simulink model "Task5AM"  (R2024a)
settings: Solver=VariableStepAuto  StartTime=0.0  StopTime=30  RelTol=1e-3
libraries: commanapbnd3 x1
settings Model: Creator=17760  LastModifiedBy=17760

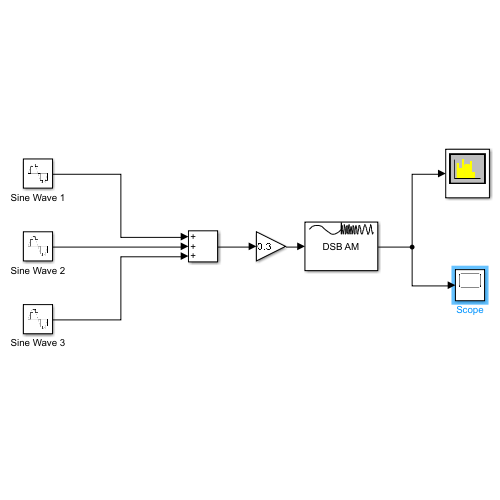
[thumbnail: Simulink's stored preview of the top-level diagram]
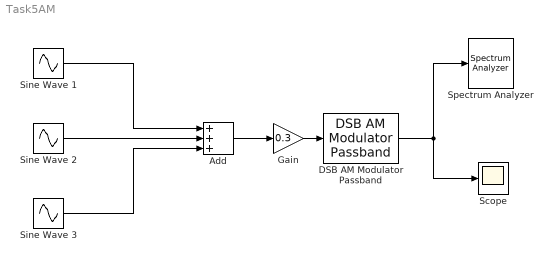
== system Task5AM ==
  Add : Sum  Inputs=+++
  DSB AM Modulator Passband : commanapbnd3/DSB AM Modulator Passband  Fc=300  Ph=0  Offset=1
  Gain : Gain  Gain=0.3
  Scope : Scope
  Sine Wave 1 : Sin  Amplitude=0.3  Frequency=2*pi*10  SampleTime=1/3000
  Sine Wave 2 : Sin  Amplitude=0.2  Frequency=2*pi*20  Phase=pi/6  SampleTime=1/3000
  Sine Wave 3 : Sin  Amplitude=0.5  Frequency=2*pi*30  Phase=pi/3  SampleTime=1/3000
  Spectrum Analyzer : SpectrumAnalyzer  WindowPosition=[1.000000,49.000000,1440.000000,889.000000,]  ScopeFrameLocation=window  YLimits=[-79.99920198,33.83925907]
  wires:
  Sine Wave 1/1 -> Add/1
  Sine Wave 2/1 -> Add/2
  Sine Wave 3/1 -> Add/3
  Add/1 -> Gain/1
  Gain/1 -> DSB AM Modulator Passband/1
  DSB AM Modulator Passband/1 -> Spectrum Analyzer/1, Scope/1
